simulink model "Marine_LocoMotive_UAV"  (R2018a)
settings: Solver=ode4  StartTime=0.0  StopTime=80  FixedStep=T  RelTol=1e-3
values from neighbouring files (symbols this model uses):
  a_11 = 0.05*m_b    (= 0.625)    [Marine_LocoMotive_UAV.m]
  a_33 = m_b    (= 12.5)    [Marine_LocoMotive_UAV.m]
  A_w = 1*1.5/2    (= 0.75)    [Marine_LocoMotive_UAV.m]
  A_w2 = 1*0.27/2    (= 0.135)    [Marine_LocoMotive_UAV.m]
  Ac = 0.0331    [Marine_LocoMotive_UAV.m]
  alpha_bar = pi/4    (= 0.785398163397)    [Marine_LocoMotive_UAV.m]
  Am = sysd.denominator{1}    [Marine_LocoMotive_UAV.m]
  Am1_LPF = sysd.denominator{1}    [Marine_LocoMotive_UAV.m]
  Am2_LPF = sysd.denominator{1}    [Marine_LocoMotive_UAV.m]
  Am_asw_LPF = sysd.denominator{1}    [Marine_LocoMotive_UAV.m]
  Am_coup_LPF = sysd.denominator{1}    [Marine_LocoMotive_UAV.m]
  Am_rdeL_LPF = sysd.denominator{1}    [Marine_LocoMotive_UAV.m]
  Am_reL_LPF = sysd.denominator{1}    [Marine_LocoMotive_UAV.m]
  Am_rref20_LPF = sysd.denominator{1}    [Marine_LocoMotive_UAV.m]
  Am_rref_LPF = sysd.denominator{1}    [Marine_LocoMotive_UAV.m]
  AmAlpha_LPF = sysd.denominator{1}    [Marine_LocoMotive_UAV.m]
  Amp_sf = 3    [Marine_LocoMotive_UAV.m]
  AmV_LPF = sysd.denominator{1}    [Marine_LocoMotive_UAV.m]
  AmZ_LPF = sysd.denominator{1}    [Marine_LocoMotive_UAV.m]
  b_11 = 0    [Marine_LocoMotive_UAV.m]
  b_33 = 2*m_b*omega_h    (= 27.5578302946)    [Marine_LocoMotive_UAV.m]
  Bm = sysd.numerator{1}    [Marine_LocoMotive_UAV.m]
  Bm1_LPF = sysd.numerator{1}    [Marine_LocoMotive_UAV.m]
  Bm2_LPF = sysd.numerator{1}    [Marine_LocoMotive_UAV.m]
  Bm_asw_LPF = sysd.numerator{1}    [Marine_LocoMotive_UAV.m]
  Bm_coup_LPF = sysd.numerator{1}    [Marine_LocoMotive_UAV.m]
  Bm_rdeL_LPF = sysd.numerator{1}    [Marine_LocoMotive_UAV.m]
  Bm_reL_LPF = sysd.numerator{1}    [Marine_LocoMotive_UAV.m]
  Bm_rref20_LPF = sysd.numerator{1}    [Marine_LocoMotive_UAV.m]
  Bm_rref_LPF = sysd.numerator{1}    [Marine_LocoMotive_UAV.m]
  BmAlpha_LPF = sysd.numerator{1}    [Marine_LocoMotive_UAV.m]
  BmV_LPF = sysd.numerator{1}    [Marine_LocoMotive_UAV.m]
  BmZ_LPF = sysd.numerator{1}    [Marine_LocoMotive_UAV.m]
  C_S = [5;9]*10^-3    [Marine_LocoMotive_UAV.m]
  Cd_u = 0.2    [Marine_LocoMotive_UAV.m]
  D_x = b_11 + D_s(1)    [Marine_LocoMotive_UAV.m]
  D_z = b_33 + D_s(2)    [Marine_LocoMotive_UAV.m]
  dc_M_p = 6.7    [Marine_LocoMotive_UAV.m]
  Delta_h = (A_im/A_b-0.5)*h_b    (= -0.0625)    [Marine_LocoMotive_UAV.m]
  eps_V = 0.1    [Marine_LocoMotive_UAV.m]
  epsilon_1 = 5    [Marine_LocoMotive_UAV.m]
  epsilon_e_u1 = 0.05    [Marine_LocoMotive_UAV.m]
  epsilon_w = 0    [Marine_LocoMotive_UAV.m]
  epsilon_w2 = pi    (= 3.14159265359)    [Marine_LocoMotive_UAV.m]
  g = 9.81    [Marine_LocoMotive_UAV.m]
  gamma_d_p = (2*0.3/0.03*2*0.2*12/4)/10    (= 2.4)    [Marine_LocoMotive_UAV.m]
  H = 10    [Marine_LocoMotive_UAV.m]
  h_b = 0.25    [Marine_LocoMotive_UAV.m]
  J_b = m_b*h_b*l_b/12    (= 0.208333333333)    [Marine_LocoMotive_UAV.m]
  J_u = 0.03    [Marine_LocoMotive_UAV.m]
  K = 40    [Marine_LocoMotive_UAV.m]
  k3 = 24    [Marine_LocoMotive_UAV.m]
  k4 = 0.8    [Marine_LocoMotive_UAV.m]
  k_w = omega_w^2/g    (= 0.123862835563)    [Marine_LocoMotive_UAV.m]
  k_w2 = omega_w2^2/g    (= 0.447144836384)    [Marine_LocoMotive_UAV.m]
  kd_a = 5.6    [Marine_LocoMotive_UAV.m]
  kd_r = 19.5    [Marine_LocoMotive_UAV.m]
  kd_t = 10    [Marine_LocoMotive_UAV.m]
  kd_x = 5    [Marine_LocoMotive_UAV.m]
  kd_z = 2    [Marine_LocoMotive_UAV.m]
  ki_a = 1.6    [Marine_LocoMotive_UAV.m]
  ki_r = 9    [Marine_LocoMotive_UAV.m]
  ki_T = 12    [Marine_LocoMotive_UAV.m]
  ki_x = 1.2    [Marine_LocoMotive_UAV.m]
  ki_z = 1    [Marine_LocoMotive_UAV.m]
  kp_a = 9.6    [Marine_LocoMotive_UAV.m]
  kp_r = 45    [Marine_LocoMotive_UAV.m]
  kp_t = 20    [Marine_LocoMotive_UAV.m]
  kp_T = 25    [Marine_LocoMotive_UAV.m]
  kp_x = 7    [Marine_LocoMotive_UAV.m]
  kp_z = 3    [Marine_LocoMotive_UAV.m]
  L = 0.2    [Marine_LocoMotive_UAV.m]
  l_b = 0.8    [Marine_LocoMotive_UAV.m]
  Lc_0 = 7    [Marine_LocoMotive_UAV.m]
  LIMIT_CMD_PITCH = 45*pi/180    (= 0.785398163397)    [Marine_LocoMotive_UAV.m]
  LIMIT_uCMD_HEIGHT = 3.5*K    (= 140)    [Marine_LocoMotive_UAV.m]
  m_b = rho_w*Vol_b/4    (= 12.5)    [Marine_LocoMotive_UAV.m]
  m_u = 1.8    [Marine_LocoMotive_UAV.m]
  min_sf = 5    [Marine_LocoMotive_UAV.m]
  nu_w = 1.787*10^-6    (= 1.787e-06)    [Marine_LocoMotive_UAV.m]
  omega_w = 2*pi/T_w    (= 1.10231321179)    [Marine_LocoMotive_UAV.m]
  omega_w2 = 2*pi/T_w2    (= 2.09439510239)    [Marine_LocoMotive_UAV.m]
  r_0 = sqrt( (X0_b(1) - X0_u(1))^2 +(X0_b(2) - X0_u(2))^2 )    [Marine_LocoMotive_UAV.m]
  r_bar = Lc_0-0.3    (= 6.7)    [Marine_LocoMotive_UAV.m]
  r_min = (zu_bar-H)-0.2    [Marine_LocoMotive_UAV.m]
  rho_a = 1.225    [Marine_LocoMotive_UAV.m]
  rho_w = 1000    [Marine_LocoMotive_UAV.m]
  T = 1/500    (= 0.002)    [Marine_LocoMotive_UAV.m]
  T_init = 10    [Marine_LocoMotive_UAV.m]
  Theta0 = 0*atan2(V_bar*D_x*cos(alpha_bar_0),V_bar*D_x*sin(alpha_bar_0)+m_u*g*cos(alpha_bar_0))    [Marine_LocoMotive_UAV.m]
  u_s = w_dir*A_w^2*omega_w*k_w*exp(2*k_w*(-Delta_h/2))    [Marine_LocoMotive_UAV.m]
  u_s2 = w_dir2*A_w2^2*omega_w2*k_w2*exp(2*k_w2*(-Delta_h/2))    [Marine_LocoMotive_UAV.m]
  u_t = -1*0.5*1    (= -0.5)    [Marine_LocoMotive_UAV.m]
  u_w = 0*0.2    (= 0)    [Marine_LocoMotive_UAV.m]
  V0_b = [u_t+u_w+u_s+v_x_w, v_z_w]    [Marine_LocoMotive_UAV.m]
  V0_u = [0 0]    [Marine_LocoMotive_UAV.m]
  V_bar = 4    [Marine_LocoMotive_UAV.m]
  Vol_b = A_b*l_b    (= 0.05)    [Marine_LocoMotive_UAV.m]
  w_dir = 1    [Marine_LocoMotive_UAV.m]
  w_dir2 = 1    [Marine_LocoMotive_UAV.m]
  X0_b = [0,H-Delta_h]    [Marine_LocoMotive_UAV.m]
  X0_u = X0_b + [3 3]    [Marine_LocoMotive_UAV.m]
  zu_bar = X0_b(2) + Lc_0*sin(alpha_bar_0)    [Marine_LocoMotive_UAV.m]
undefined symbols (not defined in the file or in its folder): Am_HPF, Am_LPF, Am_LPF2, an1, an1_v, an2, an3, Bm_HPF, Bm_LPF, Bm_LPF2, bn1, bn1_v, bn2, bn3, DiscIntNeverNeededParam, F, Light, magnitude, MIL, OMEGA_FILTER_OUTER, R_b, Tc, Tg, Tn, Ts, Tsc, Tz, X_GPS_offset
libraries: simulink x50, simulink_extras x9, aerolibwind2 x2
(part 4 of 6)

== system Marine_LocoMotive_UAV/Quadrotor+buoy/3-DOF equations of motion Earth frame/M_12 ==
  theta : Inport
  Bias : Bias
  Bias1 : Bias
  Signal Specification1 : SignalSpecification  Dimensions=2
  Signal Specification2 : SignalSpecification  Dimensions=2
  Vector Concatenate1 : Concatenate  Mode=Multidimensional array  ConcatenateDimension=2
  Vector Concatenate2 : Concatenate
  Vector Concatenate3 : Concatenate
  added mass : Subsystem
  M_12 : Outport
  wires:
  Signal Specification2/1 -> Vector Concatenate1/2
  Signal Specification1/1 -> Vector Concatenate1/1
  Vector Concatenate1/1 -> M_12/1
  Bias1/1 -> Vector Concatenate3/2
  Bias/1 -> Vector Concatenate2/1
  added mass/2(M22_I) -> Bias1/1
  added mass/3(M12_I) -> Vector Concatenate2/2, Vector Concatenate3/1
  Vector Concatenate2/1 -> Signal Specification1/1
  added mass/1(M11_I) -> Bias/1
  Vector Concatenate3/1 -> Signal Specification2/1
  theta/1 -> added mass/1(theta)

== system Marine_LocoMotive_UAV/Quadrotor+buoy/3-DOF equations of motion Earth frame/M_123 ==
  theta : Inport
  alpha : Inport  Port=2
  coupled : Inport  Port=3
  Constant1 : Constant  Value=m_u*L^2
  Constant2 : Constant  Value=m_u
  Gain : Gain  Gain=-L
  Gain1 : Gain  Gain=L
  Gain2 : Gain  Gain=L^2
  Product : Product
  Product1 : Product
  Product2 : Product
  Signal Specification1 : SignalSpecification  Dimensions=3
  Signal Specification2 : SignalSpecification  Dimensions=3
  Signal Specification3 : SignalSpecification  Dimensions=3
  Sum : Sum  Inputs=++|
  Sum1 : Sum  Inputs=++|
  Switch : Switch  Criteria=u2 > Threshold
  T, r,xu,xb{1..7} (7 alike) : Scope
  Trigonometric Function : Trigonometry  Operator=sincos
  Vector Concatenate1 : Concatenate  NumInputs=3  Mode=Multidimensional array  ConcatenateDimension=2
  Vector Concatenate2 : Concatenate  NumInputs=3
  Vector Concatenate3 : Concatenate  NumInputs=3
  Vector Concatenate4 : Concatenate  NumInputs=3
  buoy inertia : Subsystem
  M_123 : Outport
  wires:
  theta/1 -> buoy inertia/1(theta)
  Vector Concatenate3/1 -> Signal Specification2/1
  buoy inertia/1(M11_I) -> Sum/2
  Vector Concatenate2/1 -> "T, r,xu,xb7"/1, Signal Specification1/1
  Vector Concatenate4/1 -> "T, r,xu,xb6"/1, Signal Specification3/1
  buoy inertia/3(M12_I) -> Vector Concatenate2/2, Vector Concatenate3/1
  Gain/1 -> "T, r,xu,xb3"/1, Vector Concatenate4/1, Vector Concatenate2/3
  buoy inertia/2(M22_I) -> Sum1/2
  Sum/1 -> Vector Concatenate2/1
  Sum1/1 -> Vector Concatenate3/2
  alpha/1 -> Trigonometric Function/1
  Product1/1 -> Gain/1
  Product2/1 -> Gain1/1
  Switch/1 -> "T, r,xu,xb5"/1, Vector Concatenate4/3
  Vector Concatenate1/1 -> M_123/1
  Signal Specification1/1 -> Vector Concatenate1/1
  Signal Specification2/1 -> Vector Concatenate1/2
  Signal Specification3/1 -> Vector Concatenate1/3
  coupled/1 -> Switch/2, Product/2, "T, r,xu,xb1"/1
  Constant2/1 -> Product/1
  Trigonometric Function/1 -> Product1/2
  Trigonometric Function/2 -> Product2/2
  Gain1/1 -> "T, r,xu,xb4"/1, Vector Concatenate4/2, Vector Concatenate3/3
  Product/1 -> Gain2/1, Product2/1, Product1/1, "T, r,xu,xb2"/1, Sum/1, Sum1/1
  Gain2/1 -> Switch/1
  Constant1/1 -> Switch/3

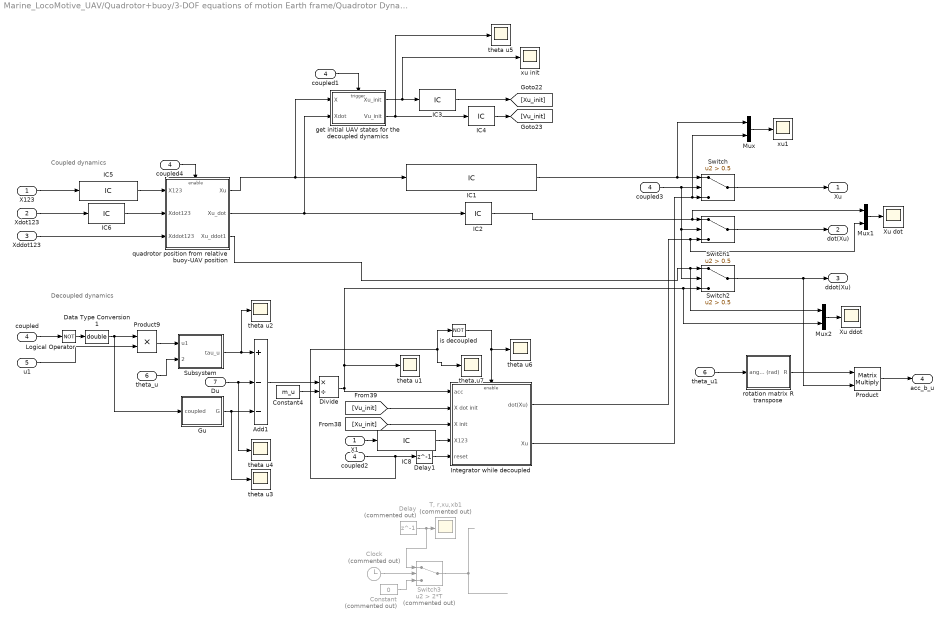
== system Marine_LocoMotive_UAV/Quadrotor+buoy/3-DOF equations of motion Earth frame/Quadrotor Dynamics Outer-Loop ==
  note: Decoupled dynamics
  note: Coupled dynamics
  X123 : Inport
  Xdot123 : Inport  Port=2
  Xddot123 : Inport  Port=3
  coupled : Inport  Port=4
  u1 : Inport  Port=5
  theta_u : Inport  Port=6
  Du : Inport  Port=7
  Add1 : Sum  Inputs=+--
  Clock : Clock  Commented=on
  Constant : Constant  Commented=on  Value=0
  Constant4 : Constant  Value=m_u
  Data Type Conversion1 : DataTypeConversion  OutDataTypeStr=double
  Delay : Delay  Commented=on  DelayLength=1
  Delay1 : Delay  DelayLength=1
  Divide : Product  Inputs=*/
  Gu : Subsystem
  IC1 : InitialCondition  Value=pos_b_ini+L*[cos(alpha_0) sin(alpha_0)]
  IC2 : InitialCondition  Value=[0 0]
  IC3 : InitialCondition  Value=X0_u
  IC4 : InitialCondition  Value=[0 0]
  IC5 : InitialCondition  Value=[X0_b alpha_bar]
  IC6 : InitialCondition  Value=[v_b_ini 0]
  IC8 : InitialCondition  Value=[X0_b alpha_bar]
  Integrator while decoupled : Subsystem  TreatAsAtomicUnit=on
  Logical Operator : Logic  Operator=NOT  AllPortsSameDT=off
  Mux : Mux  Inputs=2
  Mux1 : Mux  Inputs=2
  Mux2 : Mux  Inputs=2
  Product : Product  Multiplication=Matrix(*)
  Product9 : Product  Inputs=**  SaturateOnIntegerOverflow=on  InputSameDT=on  OutDataTypeStr=Inherit: Same as first input
  Subsystem : Subsystem
  Switch : Switch  Criteria=u2 > Threshold  Threshold=0.5
  Switch1 : Switch  Criteria=u2 > Threshold  Threshold=0.5
  Switch2 : Switch  Criteria=u2 > Threshold  Threshold=0.5
  Switch3 : Switch  Commented=on  Criteria=u2 > Threshold  Threshold=2*T
  "T, r,xu,xb1" : Scope  Commented=on
  X1 : InportShadow
  "Xu ddot  " : Scope
  "Xu dot " : Scope
  coupled{1..4} (4 alike) : InportShadow  Port=4
  get initial UAV states for the decoupled dynamics : Subsystem  TreatAsAtomicUnit=on
  is decoupled : Logic  Operator=NOT  AllPortsSameDT=off
  quadrotor position from relative buoy-UAV position : Subsystem
  rotation matrix R transpose : Subsystem
  theta u{1..7} (7 alike) : Scope
  theta_u1 : InportShadow  Port=6
  xu init : Scope
  xu1 : Scope
  Xu : Outport
  dot(Xu) : Outport  Port=2
  ddot(Xu) : Outport  Port=3
  acc_b_u : Outport  Port=4
  wires:
  Subsystem/1(tau_u) -> theta u2/1, Add1/1
  Product9/1 -> Subsystem/1(u1)
  Gu/1(G) -> theta u3/1, Add1/3
  X123/1 -> IC5/1
  Data Type Conversion1/1 -> Product9/1, Gu/1(coupled)
  Add1/1 -> Divide/1
  Logical Operator/1 -> Data Type Conversion1/1
  get initial UAV states for the decoupled dynamics/1(Xu_init) -> xu init/1, IC3/1
  get initial UAV states for the decoupled dynamics/2(Vu_init) -> IC4/1, theta u5/1
  Constant4/1 -> Divide/2
  theta_u/1 -> Subsystem/2(theta_u)
  coupled1/1 -> get initial UAV states for the decoupled dynamics/Trigger
  Du/1 -> Add1/2, theta u4/1
  coupled/1 -> Logical Operator/1
  u1/1 -> Product9/2
  coupled3/1 -> Switch2/2, Switch1/2, Switch/2
  Integrator while decoupled/2("Xu ") -> Mux/2, Switch/3
  quadrotor position from relative buoy-UAV position/1(Xu) -> IC1/1, get initial UAV states for the decoupled dynamics/1(X)
  Mux/1 -> xu1/1
  Mux1/1 -> "Xu dot "/1
  Integrator while decoupled/1("dot(Xu) ") -> Mux1/2, Switch1/3
  Mux2/1 -> "Xu ddot  "/1
  Divide/1 -> Mux2/2, Switch2/3, theta u1/1, Integrator while decoupled/1(acc)
  Switch2/1 -> Product/2, ddot(Xu)/1
  Xdot123/1 -> IC6/1
  Xddot123/1 -> quadrotor position from relative buoy-UAV position/3(Xddot123)
  quadrotor position from relative buoy-UAV position/2(Xu_dot) -> get initial UAV states for the decoupled dynamics/2(Xdot), IC2/1
  quadrotor position from relative buoy-UAV position/3(Xu_ddot1) -> Mux2/1, Switch2/1
  is decoupled/1 -> theta u6/1, Integrator while decoupled/Enable
  coupled2/1 -> Delay1/1, is decoupled/1, theta u7/1
  Switch1/1 -> dot(Xu)/1
  coupled4/1 -> quadrotor position from relative buoy-UAV position/Enable
  Switch/1 -> Xu/1
  Constant/1 -> Switch3/3
  ? -> Delay/1
  Switch3/1 -> ?
  Delay/1 -> Switch3/1, "T, r,xu,xb1"/1
  Clock/1 -> Switch3/2
  [Vu_init] -> Integrator while decoupled/2(X dot init)
  [Xu_init] -> Integrator while decoupled/3(X init)
  X1/1 -> IC8/1
  Delay1/1 -> Integrator while decoupled/5(reset)
  IC3/1 -> [Xu_init]
  IC4/1 -> [Vu_init]
  IC1/1 -> Mux/1, Switch/1
  IC2/1 -> Mux1/1, Switch1/1
  IC5/1 -> quadrotor position from relative buoy-UAV position/1(X123)
  IC8/1 -> Integrator while decoupled/4(X123)
  IC6/1 -> quadrotor position from relative buoy-UAV position/2(Xdot123)
  theta_u1/1 -> rotation matrix R transpose/1(angle (rad))
  rotation matrix R transpose/1(R) -> Product/1
  Product/1 -> acc_b_u/1

== system Marine_LocoMotive_UAV/Quadrotor+buoy/3-DOF equations of motion Earth frame/Tension from Buoy, X direction ==
  alpha : Inport
  M12 : Inport  Port=2
  D12 : Inport  Port=3
  Vr,Wr : Inport  Port=4
  Xb_ddot : Inport  Port=5
  G : Inport  Port=6
  FB : Inport  Port=7
  Add1 : Sum  Inputs=+++-
  Constant : Constant  Value=0
  Math Function : Math  Operator=reciprocal  SaturateOnIntegerOverflow=on
  Math Function1 : Math  Operator=reciprocal  SaturateOnIntegerOverflow=on
  Product1 : Product
  Product2 : Product  Inputs=**  Multiplication=Matrix(*)
  Product3 : Product  Inputs=**  Multiplication=Matrix(*)
  Scope5 : Scope
  Trigonometric Function3 : Trigonometry  Operator=sincos
  Vector Concatenate2 : Concatenate
  Vector Concatenate3 : Concatenate
  T x,z : Outport
  wires:
  alpha/1 -> Trigonometric Function3/1
  M12/1 -> Product2/1
  Vr,Wr/1 -> Product3/2
  D12/1 -> Product3/1
  Xb_ddot/1 -> Product2/2
  G/1 -> Add1/3
  Product2/1 -> Add1/2
  Trigonometric Function3/2 -> Math Function/1
  Trigonometric Function3/1 -> Math Function1/1
  Product3/1 -> Add1/1
  Math Function/1 -> Vector Concatenate2/1
  Math Function1/1 -> Vector Concatenate2/2
  Constant/1 -> Vector Concatenate3/1
  Vector Concatenate3/1 -> Add1/4
  FB/1 -> Vector Concatenate3/2
  Product1/1 -> Scope5/1, T x,z/1
  Vector Concatenate2/1 -> Product1/2
  Add1/1 -> Product1/1

== system Marine_LocoMotive_UAV/Quadrotor+buoy/3-DOF equations of motion Earth frame/Tension from UAV, X and r directions ==
  alpha : Inport
  r_p_ddot : Inport  Port=2
  theta_u : Inport  Port=3
  u1 : Inport  Port=4
  Xb_ddot : Inport  Port=5
  Xu_ddot : Inport  Port=6
  Add1 : Sum  Inputs=+-+
  Add2 : Sum  Inputs=---
  Add3 : Sum  Commented=on  Inputs=+-
  Discrete Derivative2 : simulink/Discrete/Discrete Derivative  Commented=on  gainval=1.0  ICPrevScaledInput=L*500  OutMin=[]  OutMax=[]  OutDataType=fixdt(1, 16)  OutScaling=2^-10  DoSatur=off
  Discrete Derivative3 : simulink/Discrete/Discrete Derivative  Commented=on  gainval=1.0  ICPrevScaledInput=0  OutMin=[]  OutMax=[]  OutDataType=fixdt(1, 16)  OutScaling=2^-10  DoSatur=off
  Gain14 : Gain  Commented=on
  Gain15 : Gain  Commented=on  Gain=m_u
  Gain5 : Gain  Gain=m_u
  Gain6 : Gain  Gain=m_u*g
  Product10 : Product  Inputs=**  Multiplication=Matrix(*)
  Product12 : Product  Commented=on
  Product7 : Product
  Product9 : Product  Commented=on  Inputs=*/
  Signal Specification{1,4..6} (4 alike) : SignalSpecification  Dimensions=1
  Signal Specification2 : SignalSpecification  Dimensions=[1,2]
  Sum4 : Sum  Inputs=|++
  "T, r,xu,xb1" : Scope
  "T, r,xu,xb2" : Scope
  "T, r,xu,xb3" : Scope
  "Tension from UAV, X and r directions" : Subsystem
  Trigonometric Function2 : Trigonometry
  Trigonometric Function3 : Trigonometry  Operator=sincos
  Trigonometric Function6 : Trigonometry  Commented=on  Operator=cos
  Trigonometric Function8 : Trigonometry  Commented=on
  Vector Concatenate : Concatenate
  Xu_ddot1 : InportShadow  Port=6
  alpha1 : InportShadow
  r : Constant  Commented=on  Value=L
  theta_u1 : InportShadow  Port=3
  "u1 " : InportShadow  Port=4
  x_ddot1 : Selector  Commented=on  InputPortWidth=2  IndexOptions=Index vector (dialog)  Indices=1  OutputSizes=1
  "T, from r" : Outport
  "T, from uav z" : Outport  Port=2
  wires:
  r/1 -> Discrete Derivative2/1
  r_p_ddot/1 -> Add2/1
  alpha/1 -> Trigonometric Function3/1
  Sum4/1 -> Trigonometric Function2/1
  [alpha] -> Sum4/1
  u1/1 -> Product7/2
  Add2/1 -> Gain5/1
  Trigonometric Function2/1 -> Product7/1
  Discrete Derivative2/1 -> Discrete Derivative3/1
  Trigonometric Function3/1 -> Signal Specification5/1, Vector Concatenate/2
  Product10/1 -> Add2/2
  Gain5/1 -> "T, r,xu,xb1"/1, Add1/1
  theta_u/1 -> Sum4/2
  Gain6/1 -> "T, r,xu,xb2"/1, Add1/2
  Trigonometric Function3/2 -> Vector Concatenate/1
  Add3/1 -> Product9/1
  Gain14/1 -> Add3/1
  Trigonometric Function8/1 -> Product12/1
  "u1 "/1 -> "Tension from UAV, X and r directions"/3(u1), Product12/2
  alpha1/1 -> "Tension from UAV, X and r directions"/1(alpha), Trigonometric Function6/1
  Product12/1 -> Gain14/1
  x_ddot1/1 -> Gain15/1
  Trigonometric Function6/1 -> Product9/2
  Xu_ddot/1 -> x_ddot1/1
  theta_u1/1 -> "Tension from UAV, X and r directions"/2(theta_u), Trigonometric Function8/1
  Gain15/1 -> Add3/2
  Product7/1 -> Signal Specification6/1
  Signal Specification2/1 -> Product10/1
  Discrete Derivative3/1 -> Signal Specification4/1
  Add1/1 -> Signal Specification1/1
  Vector Concatenate/1 -> Product10/2
  Signal Specification4/1 -> Add2/3
  Signal Specification5/1 -> Gain6/1
  Signal Specification6/1 -> "T, r,xu,xb3"/1, Add1/3
  Xb_ddot/1 -> Signal Specification2/1
  Signal Specification1/1 -> "T, from r"/1
  Xu_ddot1/1 -> "Tension from UAV, X and r directions"/4(Xu_ddot)
  "Tension from UAV, X and r directions"/1("T, from x simple") -> "T, from uav z"/1

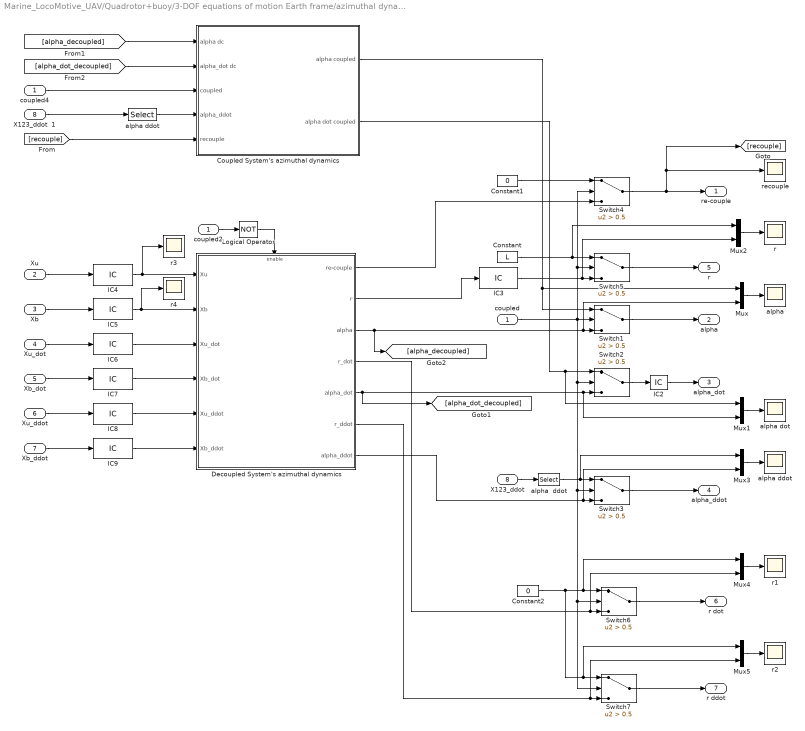
== system Marine_LocoMotive_UAV/Quadrotor+buoy/3-DOF equations of motion Earth frame/azimuthal dynamics ==
  coupled : Inport
  Xu : Inport  Port=2
  Xb : Inport  Port=3
  "Xu_dot " : Inport  Port=4
  Xb_dot : Inport  Port=5
  Xu_ddot : Inport  Port=6
  "Xb_ddot   " : Inport  Port=7
  "X123_ddot  " : Inport  Port=8
  "    alpha ddot" : Scope
  "  alpha" : Scope
  "  alpha dot" : Scope
    r{,1..4} (5 alike) : Scope
  "  recouple   " : Scope
  Constant : Constant  Value=L
  Constant1 : Constant  Value=0
  Constant2 : Constant  Value=0
  Coupled System's azimuthal dynamics : Subsystem
  Decoupled System's azimuthal dynamics : Subsystem  TreatAsAtomicUnit=on
  IC2 : InitialCondition  Value=0
  IC3 : InitialCondition  Value=r_0
  IC4 : InitialCondition  Value=X0_u
  IC5 : InitialCondition  Value=X0_b
  IC6 : InitialCondition  Value=[0 0]
  IC7 : InitialCondition  Value=V0_b
  IC8 : InitialCondition  Value=[0 0]
  IC9 : InitialCondition  Value=[0 0]
  Logical Operator : Logic  Operator=NOT  AllPortsSameDT=off  OutDataTypeStr=boolean
  Mux{,1..5} (6 alike) : Mux  Inputs=2
  Switch{1..7} (7 alike) : Switch  Criteria=u2 > Threshold  Threshold=0.5
  X123_ddot  1 : InportShadow  Port=8
  alpha  ddot : Selector  InputPortWidth=3  IndexOptions=Index vector (dialog)  Indices=3  OutputSizes=1
  alpha ddot : Selector  InputPortWidth=3  IndexOptions=Index vector (dialog)  Indices=3  OutputSizes=1
  coupled2 : InportShadow
  coupled4 : InportShadow
  re-couple : Outport
  alpha : Outport  Port=2
  "alpha_dot " : Outport  Port=3
  alpha_ddot : Outport  Port=4
  "r " : Outport  Port=5
  r dot : Outport  Port=6
  r ddot : Outport  Port=7
  wires:
  coupled/1 -> Switch7/2, Switch6/2, Switch3/2, Switch2/2, Switch4/2, Switch5/2, Switch1/2
  "X123_ddot  "/1 -> alpha  ddot/1
  Switch3/1 -> alpha_ddot/1
  Coupled System's azimuthal dynamics/2(alpha dot coupled) -> Switch2/1, Mux1/1
  Switch2/1 -> IC2/1
  Xb/1 -> IC5/1
  Xu/1 -> IC4/1
  alpha ddot/1 -> Coupled System's azimuthal dynamics/4(alpha_ddot)
  [alpha_dot_decoupled] -> Coupled System's azimuthal dynamics/2(alpha_dot dc)
  coupled4/1 -> Coupled System's azimuthal dynamics/3(coupled)
  [alpha_decoupled] -> Coupled System's azimuthal dynamics/1(alpha dc)
  X123_ddot  1/1 -> alpha ddot/1
  "Xu_dot "/1 -> IC6/1
  Xb_dot/1 -> IC7/1
  "Xb_ddot   "/1 -> IC9/1
  Xu_ddot/1 -> IC8/1
  coupled2/1 -> Logical Operator/1
  Switch5/1 -> "r "/1
  Constant/1 -> Switch5/1, Mux2/1
  Decoupled System's azimuthal dynamics/2(r) -> IC3/1
  [recouple] -> Coupled System's azimuthal dynamics/5(recouple)
  Coupled System's azimuthal dynamics/1(alpha coupled) -> Mux/1, Switch1/1
  Decoupled System's azimuthal dynamics/7(alpha_ddot) -> Mux3/2, Switch3/3
  Logical Operator/1 -> Decoupled System's azimuthal dynamics/Enable
  Mux/1 -> "  alpha"/1
  Mux1/1 -> "  alpha dot"/1
  Decoupled System's azimuthal dynamics/5(alpha_dot) -> Mux1/2, Switch2/3, [alpha_dot_decoupled]
  Mux2/1 -> "  r"/1
  Decoupled System's azimuthal dynamics/1(re-couple) -> Switch4/3
  Mux3/1 -> "    alpha ddot"/1
  alpha  ddot/1 -> Mux3/1, Switch3/1
  Switch4/1 -> [recouple], "  recouple   "/1, re-couple/1
  Constant1/1 -> Switch4/1
  Switch1/1 -> alpha/1
  IC2/1 -> "alpha_dot "/1
  Mux4/1 -> "  r1"/1
  Switch6/1 -> r dot/1
  Decoupled System's azimuthal dynamics/4(r_dot) -> Mux4/2, Switch6/3
  Decoupled System's azimuthal dynamics/6(r_ddot) -> Switch7/3, Mux5/2
  Constant2/1 -> Switch7/1, Mux5/1, Mux4/1, Switch6/1
  Switch7/1 -> r ddot/1
  Mux5/1 -> "  r2"/1
  IC3/1 -> Mux2/2, Switch5/3
  IC4/1 -> "  r3"/1, Decoupled System's azimuthal dynamics/1(Xu)
  IC6/1 -> Decoupled System's azimuthal dynamics/3(Xu_dot)
  IC7/1 -> Decoupled System's azimuthal dynamics/4(Xb_dot)
  IC8/1 -> Decoupled System's azimuthal dynamics/5(Xu_ddot)
  IC9/1 -> Decoupled System's azimuthal dynamics/6(Xb_ddot)
  Decoupled System's azimuthal dynamics/3(alpha) -> Switch1/3, Mux/2, [alpha_decoupled]
  IC5/1 -> "  r4"/1, Decoupled System's azimuthal dynamics/2(Xb)

== system Marine_LocoMotive_UAV/Quadrotor+buoy/3-DOF equations of motion Earth frame/buoyancy ==
  z_b : Inport
  zeta : Inport  Port=2
  Constant : Constant  Commented=on  Value=g*rho_w*l_b*R_b
  Manual Switch : ManualSwitch  CurrentSetting=0
  Product : Product  Commented=on
  Scope1 : Scope  Commented=on
  Scope3 : Scope  Commented=on
  V_im cuboid : Subsystem
  f(z_b,zeta) cylinder : Subsystem  Commented=on
  two connected cylindrical buoys : Gain  Commented=on  Gain=2
  two connected cylindrical buoys1 : Gain  Commented=on  Gain=l_b*R_b
  two connected cylindrical buoys2 : Gain  Commented=on  Gain=2
  V_im : Outport
  wires:
  z_b/1 -> V_im cuboid/2(zb), f(z_b,zeta) cylinder/2(zb)
  zeta/1 -> V_im cuboid/1(zeta), f(z_b,zeta) cylinder/1(zeta)
  Product/1 -> two connected cylindrical buoys/1
  Constant/1 -> Scope1/1, Product/2
  f(z_b,zeta) cylinder/1(Out1) -> two connected cylindrical buoys1/1, Product/1, Scope3/1
  Manual Switch/1 -> V_im/1
  V_im cuboid/1(Vol_im) -> Manual Switch/2
  two connected cylindrical buoys1/1 -> two connected cylindrical buoys2/1
  two connected cylindrical buoys2/1 -> Manual Switch/1

== system Marine_LocoMotive_UAV/Quadrotor+buoy/3-DOF equations of motion Earth frame/rotation matrix R  ==
  angle (rad) : Inport
  Gain : Gain  Gain=-1
  Signal Specification1 : SignalSpecification  Dimensions=2
  Signal Specification2 : SignalSpecification  Dimensions=2
  Trigonometric Function1 : Trigonometry  Operator=sincos
  Vector Concatenate1 : Concatenate  Mode=Multidimensional array  ConcatenateDimension=2
  Vector Concatenate2 : Concatenate
  Vector Concatenate3 : Concatenate
  R : Outport
  wires:
  Signal Specification2/1 -> Vector Concatenate1/2
  Signal Specification1/1 -> Vector Concatenate1/1
  Vector Concatenate1/1 -> R/1
  Vector Concatenate2/1 -> Signal Specification1/1
  Vector Concatenate3/1 -> Signal Specification2/1
  angle (rad)/1 -> Trigonometric Function1/1
  Trigonometric Function1/2 -> Vector Concatenate3/2, Vector Concatenate2/1
  Trigonometric Function1/1 -> Vector Concatenate2/2, Gain/1
  Gain/1 -> Vector Concatenate3/1

== system Marine_LocoMotive_UAV/Quadrotor+buoy/3-DOF equations of motion Earth frame/u123 ==
  u1 : Inport
  theta : Inport  Port=2
  V_im : Inport  Port=3
  alpha : Inport  Port=4
  coupled : Inport  Port=5
  Constant1 : Constant  Value=rho_w*g
  Constant2 : Constant  Commented=on  Value=Vol_b/2
  F_B : Product
  Gain : Gain  Gain=L
  Product1 : Product  Inputs=3  SaturateOnIntegerOverflow=on  InputSameDT=on  OutDataTypeStr=Inherit: Same as first input
  Product2 : Product  Inputs=**  SaturateOnIntegerOverflow=on  InputSameDT=on  OutDataTypeStr=Inherit: Same as first input
  Product6 : Product  Inputs=**  SaturateOnIntegerOverflow=on  InputSameDT=on  OutDataTypeStr=Inherit: Same as first input
  Product7 : Product  Inputs=**  SaturateOnIntegerOverflow=on  InputSameDT=on  OutDataTypeStr=Inherit: Same as first input
  Scope9 : Scope
  Signal Specification2 : SignalSpecification  Dimensions=3
  Sum1 : Sum  Inputs=|++  SaturateOnIntegerOverflow=on
  Sum2 : Sum  Inputs=|++  SaturateOnIntegerOverflow=on
  Trigonometric Function1 : Trigonometry  Operator=sincos
  Trigonometric Function2 : Trigonometry  Operator=cos
  Vector Concatenate3 : Concatenate  NumInputs=3
  coupled1 : InportShadow  Port=5
  u2 : InportShadow
  u123 : Outport
  wires:
  Product7/1 -> Sum1/1
  Product2/1 -> Product7/2, Product6/1
  Trigonometric Function1/2 -> Product7/1
  Product1/1 -> Vector Concatenate3/3
  Vector Concatenate3/1 -> Scope9/1, Signal Specification2/1
  Product6/1 -> Vector Concatenate3/1
  Sum1/1 -> Vector Concatenate3/2
  Trigonometric Function1/1 -> Product6/2
  F_B/1 -> Sum1/2
  theta/1 -> Sum2/1, Trigonometric Function1/1
  V_im/1 -> F_B/1
  alpha/1 -> Sum2/2
  Sum2/1 -> Trigonometric Function2/1
  Trigonometric Function2/1 -> Gain/1
  Gain/1 -> Product1/2
  u2/1 -> Product1/1
  Constant1/1 -> F_B/2
  Signal Specification2/1 -> u123/1
  coupled/1 -> Product2/1
  u1/1 -> Product2/2
  coupled1/1 -> Product1/3

== system Marine_LocoMotive_UAV/Sensors and Filters/Coupling detection by r/Coupling state ==
  r_est : Inport
  re_couple : Inport  Port=2
  Data Type Conversion : DataTypeConversion  OutDataTypeStr=double
  Delay10 : Delay  DelayLength=1  InitialCondition=0
  IC3 : InitialCondition  Value=0
  IC5 : InitialCondition  Value=0
  MATLAB Function : MATLAB Function  TreatAsAtomicUnit=on
  "T, r,xu,xb1" : Scope
  break algebraic loop : Delay  DelayLength=1  InitialCondition=1
  cable length with safety margine1 : simulink/Logic and Bit Operations/Compare To Constant  relop=>=  const=Lc_0-0.05  OutDataTypeStr=boolean
  "is coupled " : Scope
  is coupled -1 : Scope
  pos tension : Scope
  positive tension : Scope
  "re_couple " : Scope
  state detector : Scope
  is coupled : Outport
  wires:
  Delay10/1 -> is coupled -1/1, MATLAB Function/3(coupled)
  IC5/1 -> is coupled/1, Delay10/1
  MATLAB Function/1(is_coupled) -> IC5/1, "is coupled "/1
  break algebraic loop/1 -> pos tension/1, MATLAB Function/1(pos_T)
  re_couple/1 -> MATLAB Function/2(re_couple), "re_couple "/1
  MATLAB Function/2(c) -> state detector/1
  Data Type Conversion/1 -> positive tension/1, break algebraic loop/1
  IC3/1 -> Data Type Conversion/1
  cable length with safety margine1/1 -> IC3/1
  r_est/1 -> "T, r,xu,xb1"/1, cable length with safety margine1/1

== system Marine_LocoMotive_UAV/Sensors and Filters/Data processing/Estimate Attitude ==
  Acc : Inport
  q : Inport  Port=2
  Euler : Inport  Port=3
  Calculate Roll and Pitch (From Acceleration Data) : Subsystem
  Constant : Constant  Value=Ts
  Demux : Demux  Outputs=2
  Ground : Ground
  High Pass Filter1 : DiscreteTransferFcn  Numerator=Bm_HPF  Denominator=Am_HPF
  Kalman Filter - Pitch : MATLAB Function  TreatAsAtomicUnit=on
  Manual Switch1 : ManualSwitch  CurrentSetting=0
  Mux : Mux  Inputs=3
  Mux2 : Mux  Inputs=2
  Mux5 : Mux  Inputs=2
  Notch Filter1 : Subsystem
  Scope1 : Scope
  Signal Specification : SignalSpecification  Dimensions=1
  theta : Scope
  q_g : Outport
  q_f : Outport  Port=2
  " pitch" : Outport  Port=3
  wires:
  q/1 -> High Pass Filter1/1, Mux2/2
  Notch Filter1/2(q) -> Kalman Filter - Pitch/2(gyro_rate), q_f/1
  Calculate Roll and Pitch (From Acceleration Data)/1(pitch_acc (rad)) -> Kalman Filter - Pitch/1(acc_angle)
  Signal Specification/1 -> " pitch"/1  "Kalman"
  Euler/1 -> Mux5/1, Kalman Filter - Pitch/3(opti_angle)  "pitch"
  Constant/1 -> Kalman Filter - Pitch/4(dt)
  Acc/1 -> Demux/1
  Notch Filter1/1(y) -> Manual Switch1/2
  High Pass Filter1/1 -> Manual Switch1/1, Notch Filter1/1(u), Mux2/1
  Mux2/1 -> Scope1/1
  Kalman Filter - Pitch/1(angle) -> Mux5/2, Signal Specification/1
  Mux/1 -> Calculate Roll and Pitch (From Acceleration Data)/1(accel (m/s^2) [3])
  Demux/1 -> Mux/1
  Demux/2 -> Mux/3
  Ground/1 -> Mux/2
  Manual Switch1/1 -> q_g/1
  Mux5/1 -> theta/1

== system Marine_LocoMotive_UAV/Sensors and Filters/Data processing/Estimate Position ==
  OptiTrack : Inport
  "pitch, Kalman" : Inport  Port=2
  Sonar : Inport  Port=3
  2nd Order Filter : Subsystem
  2nd Order Filter2 : Subsystem
  2nd Order Filter4 : Subsystem
  2nd Order Filter5 : Subsystem
  Constant4 : Constant  Value=Tc
  Demux2 : Demux
  Extrapolation - x : MATLAB Function  TreatAsAtomicUnit=on
  Extrapolation - z : MATLAB Function  TreatAsAtomicUnit=on
  Height est : Scope
  Height est1 : Scope
  Kalman Filter - Height : MATLAB Function  TreatAsAtomicUnit=on
  Manual Switch : ManualSwitch  CurrentSetting=0
  Mux : Mux  Inputs=2
  Mux1 : Mux  Inputs=2
  Mux2 : Mux  Inputs=3
  Mux3 : Mux  Inputs=3
  Mux4 : Mux  Inputs=3
  Notch Filter2 : Subsystem
  Position : Selector  InputPortWidth=5  IndexOptions=Index vector (dialog)  Indices=[1 2 4 5]  OutputSizes=1
  Signal Conditioning - Sonar : Subsystem
  Signal Specification : SignalSpecification  Dimensions=2
  Signal Specification1 : SignalSpecification  Dimensions=2
  Step Size : Constant  Value=Tc
  Step Size1 : Constant  Value=X0_u(1)
  Step Size2 : Constant  Value=X0_u(2)
  Step Size3 : Constant  Value=X0_u(2)
  Terminator1 : Terminator
  Terminator2 : Terminator
  Thrust1 : Scope
  Thrust11 : Scope
  V_est : Scope  Commented=on
  X_est : Scope  Commented=on
  Xe : Outport
  Ve : Outport  Port=2
  wires:
  Demux2/1 -> Mux3/1, Extrapolation - x/1(xin)
  2nd Order Filter5/2(yd) -> [height_rate_Kalman]
  Demux2/3 -> Extrapolation - x/4(new), Extrapolation - z/4(new)  "New Data"
  Constant4/1 -> Kalman Filter - Height/3(dt)
  Extrapolation - x/1(xout) -> Mux3/2, 2nd Order Filter/1(u)
  2nd Order Filter/1(y) -> Mux3/3, Mux/1
  2nd Order Filter4/2(yd) -> Kalman Filter - Height/2(sonar_d)
  2nd Order Filter2/1(y) -> Mux4/3, Kalman Filter - Height/1(optitrack), Mux2/2
  Sonar/1 -> Signal Conditioning - Sonar/1(sonar (m))
  2nd Order Filter4/1(y) -> Terminator1/1
  Signal Conditioning - Sonar/1(calib sonar (m)) -> Mux2/1, 2nd Order Filter4/1(u)
  Step Size/1 -> Extrapolation - z/3(dt), Extrapolation - x/3(dt)
  Position/1 -> Demux2/1
  Demux2/2 -> Mux4/1, Extrapolation - z/1(xin)
  2nd Order Filter5/1(y) -> Terminator2/1
  Mux/1 -> Signal Specification/1  "Xe IMU or GPS"
  [height_rate_Kalman] -> Mux1/2
  Demux2/4 -> Extrapolation - x/5(isTracking), Extrapolation - z/5(isTracking)  "Is Tracking"
  Mux2/1 -> Height est/1
  Mux1/1 -> Signal Specification1/1  "Ve IMU or GPS"
  OptiTrack/1 -> Thrust1/1, Position/1
  Mux3/1 -> Thrust11/1
  2nd Order Filter2/2(yd) -> Extrapolation - z/2(xdotin)
  Notch Filter2/1(y) -> Manual Switch/2
  2nd Order Filter/2(yd) -> Notch Filter2/1(u), Manual Switch/1, Extrapolation - x/2(xdotin)
  Manual Switch/1 -> Mux1/1
  Signal Specification/1 -> Xe/1, X_est/1
  Signal Specification1/1 -> Ve/1, V_est/1
  Kalman Filter - Height/1(height) -> [height_Kalman], Mux2/3, 2nd Order Filter5/1(u)
  [height_Kalman] -> Mux/2
  "pitch, Kalman"/1 -> Signal Conditioning - Sonar/2(pitch (rad))
  Mux4/1 -> Height est1/1
  Extrapolation - z/1(xout) -> Mux4/2, 2nd Order Filter2/1(u)
  Step Size1/1 -> Extrapolation - x/6(x0)
  Step Size2/1 -> Extrapolation - z/6(x0)
  Step Size3/1 -> Kalman Filter - Height/4(x0)

== system Marine_LocoMotive_UAV/Sensors and Filters/Sensors/ Sonar (10Hz) (true elevation instead real sonar signal) ==
  note: "Smooth" out the Sonar data
  note: Resample the 10Hz Sonar Data
  sonar (m) : Inport
  FOH1 : Subsystem  mask{Ts=0.1}
      mask prompts: Ts "Sample Time"
  IC : InitialCondition  Value=X0_u(2)
  Rate Transition : RateTransition  InitialCondition=X0_u(2)
  Sampler : Subsystem  mask{Ts=0.1}
      mask prompts: Ts "Sample Time"
  calib sonar (m) : Outport
  wires:
  Sampler/1(Out1) -> Rate Transition/1
  Rate Transition/1 -> FOH1/1(Input)
  sonar (m)/1 -> Sampler/1(In1)
  FOH1/1(Output) -> IC/1
  IC/1 -> calib sonar (m)/1

== system Marine_LocoMotive_UAV/Sensors and Filters/Sensors/Accelerometer (500Hz) ==
  Ab : Inport
  "Ab " : Scope  Commented=on
  Demux1 : Demux  Outputs=2
  From File : FromFile  FileName=acc_x_noise.mat  SampleTime=Tz
  From File2 : FromFile  FileName=acc_z_noise.mat  SampleTime=Tz
  IC : InitialCondition  Value=[0 0]
  Manual Switch{,2,4,6} (4 alike) : ManualSwitch
  Mux1 : Mux  Inputs=2
  Mux2 : Mux  Inputs=2
  Product : Product  SaturateOnIntegerOverflow=on  RndMeth=Zero  InputSameDT=on  OutDataTypeStr=Inherit: Same as first input
  Product2 : Product  SaturateOnIntegerOverflow=on  RndMeth=Zero  InputSameDT=on  OutDataTypeStr=Inherit: Same as first input
  Slider Gain : simulink/Math Operations/Slider Gain  gain=1  low=0  high=2
  Slider Gain2 : simulink/Math Operations/Slider Gain  gain=1  low=0  high=2
  Sum2 : Sum  Inputs=+++  SaturateOnIntegerOverflow=on  InputSameDT=on  OutDataTypeStr=Inherit: Same as first input
  Sum5 : Sum  Inputs=+++  SaturateOnIntegerOverflow=on  InputSameDT=on  OutDataTypeStr=Inherit: Same as first input
  acc_noisy : Scope  Commented=on
  bias : Constant  Value=0.05  VectorParams1D=off
  bias10 : Constant  Value=1.02  VectorParams1D=off
  bias11 : Constant  VectorParams1D=off
  bias3 : Constant  Value=1.02  VectorParams1D=off
  bias4 : Constant  VectorParams1D=off
  bias6 : Constant  Value=0  VectorParams1D=off
  bias7 : Constant  Value=0.05  VectorParams1D=off
  bias8 : Constant  Value=0  VectorParams1D=off
  Acc : Outport
  wires:
  bias11/1 -> Manual Switch6/2
  bias10/1 -> Manual Switch6/1
  bias4/1 -> Manual Switch4/2
  bias3/1 -> Manual Switch4/1
  Manual Switch2/1 -> Sum2/2
  bias8/1 -> Manual Switch2/2
  bias7/1 -> Manual Switch2/1
  bias6/1 -> Manual Switch/2
  bias/1 -> Manual Switch/1
  Manual Switch/1 -> Sum5/2
  Manual Switch6/1 -> Product2/1
  Manual Switch4/1 -> Product/1
  Product2/1 -> Mux1/2
  Sum2/1 -> Product2/2
  Product/1 -> Mux1/1
  Sum5/1 -> Product/2
  From File2/1 -> Slider Gain2/1
  Demux1/1 -> Sum5/3
  Demux1/2 -> Sum2/3
  From File/1 -> Slider Gain/1
  Mux2/1 -> acc_noisy/1
  Mux1/1 -> IC/1
  Ab/1 -> Demux1/1, Mux2/2, "Ab "/1
  Slider Gain/1 -> Sum5/1
  Slider Gain2/1 -> Sum2/1
  IC/1 -> Mux2/1, Acc/1

== system Marine_LocoMotive_UAV/Sensors and Filters/Sensors/GPS (10Hz)  ==
  note: 0.2
  Xe : Inport
  Euler : Inport  Port=2
  DCM_b2e : Inport  Port=3
  Constant : Constant  Value=X_GPS_offset
  Constant1 : Constant
  Demux : Demux  Outputs=2
  IC : InitialCondition  Value=[X0_u Theta0]
  Is Tracking : simulink/Sources/Repeating Sequence Stair  Commented=on  OutValues=[1 1 1 1 1 1 1 1 1 1 1 1 1 1 1 1 1 1 1 1]  tsamp=To  OutMin=[]  OutMax=[]  OutDataTypeStr=double  OutputDataTypeScalingMode=double  OutDataType=fixdt(0,8)  ConRadixGroup=Best Precision: Vector-wise  OutScaling=2^-12
  Logical Operator : Logic  AllPortsSameDT=off  OutDataTypeStr=boolean
  Mux : Mux  Inputs=3
  Mux1 : Mux  Inputs=3
  New Data : simulink/Sources/Repeating Sequence Stair  Commented=on  OutValues=[1 1 1 0 0 1 0 1 1 1 1 0 1 1 0 1 1 1 1 1 0 0 0 1 1 0 1 1 1 0]  tsamp=To  OutMin=[]  OutMax=[]  OutDataTypeStr=double  OutputDataTypeScalingMode=double  OutDataType=fixdt(0,8)  ConRadixGroup=Best Precision: Vector-wise  OutScaling=2^-12
  Product : Product  Multiplication=Matrix(*)
  Random Number : RandomNumber  Variance=5/10000  SampleTime=Tg
  Random Number2 : RandomNumber  Variance=5/10000  SampleTime=Tg
  Random Number4 : RandomNumber  Variance=1/100000  SampleTime=Tg
  Rate Transition : RateTransition
  Rate Transition2 : RateTransition
  Rate Transition4 : RateTransition
  Scope : Scope  Commented=on
  Slider Gain : simulink/Math Operations/Slider Gain  gain=0.5  low=0  high=2
  Slider Gain2 : simulink/Math Operations/Slider Gain  gain=0.5  low=0  high=2
  Slider Gain4 : simulink/Math Operations/Slider Gain  gain=1  low=0  high=2
  Sum : Sum  Inputs=++|
  Sum2 : Sum  Inputs=++|
  Sum4 : Sum  Inputs=++|
  Sum6 : Sum  Inputs=|++
  Switch : Switch  Criteria=u2 > Threshold  Threshold=0.5
  Variable Integer Delay1 : Delay  DelayLength=1
  Variable Integer Delay3 : Delay  DelayLength=1  InitialCondition=[X0_u Theta0]
  optiTrack : Scope  Commented=on
  optiTrack1 : Scope  Commented=on
  optiTrack2 : Scope
  optiTrack3 : Scope
  optiTrack4 : Scope
  GPS : Outport
  wires:
  Mux/1 -> Variable Integer Delay3/1
  Constant1/1 -> Mux1/2, Logical Operator/1, Mux1/3, Logical Operator/2
  Logical Operator/1 -> optiTrack1/1, Switch/2
  Variable Integer Delay1/1 -> Switch/3
  Slider Gain/1 -> Sum2/1
  Random Number2/1 -> Rate Transition2/1
  Demux/1 -> Sum/2
  Demux/2 -> Sum2/2
  Sum2/1 -> Mux/2
  Sum/1 -> Mux/1
  Random Number/1 -> Rate Transition/1
  Slider Gain2/1 -> optiTrack2/1, Sum/1
  Mux1/1 -> GPS/1
  Random Number4/1 -> Rate Transition4/1
  Euler/1 -> Sum4/2
  Sum4/1 -> Mux/3
  Variable Integer Delay3/1 -> Switch/1, optiTrack3/1
  Rate Transition/1 -> Slider Gain2/1
  Rate Transition2/1 -> Scope/1, Slider Gain/1
  Rate Transition4/1 -> Slider Gain4/1
  Switch/1 -> Variable Integer Delay1/1, IC/1  "x,z,theta"
  Sum6/1 -> Demux/1
  DCM_b2e/1 -> Product/1
  Constant/1 -> Product/2
  Product/1 -> Sum6/2
  Xe/1 -> Sum6/1
  IC/1 -> optiTrack/1, Mux1/1
  Slider Gain4/1 -> Sum4/1, optiTrack4/1

== system Marine_LocoMotive_UAV/Sensors and Filters/Sensors/Gyro (500Hz) ==
  q : Inport
  Degrees to Radians2 : simulink_extras/Transformations/Degrees to Radians
  From File1 : FromFile  FileName=gyro_q_noise.mat  SampleTime=Tz
  Manual Switch1 : ManualSwitch
  Manual Switch5 : ManualSwitch  CurrentSetting=0
  Product1 : Product  SaturateOnIntegerOverflow=on  RndMeth=Zero  InputSameDT=on  OutDataTypeStr=Inherit: Same as first input
  Slider Gain1 : simulink/Math Operations/Slider Gain  gain=1  low=0  high=2
  Sum2 : Sum  Inputs=+++  SaturateOnIntegerOverflow=on  InputSameDT=on  OutDataTypeStr=Inherit: Same as first input
  Variable Integer Delay3 : Delay  DelayLength=0
  bias1 : Constant  Value=-1  VectorParams1D=off
  bias2 : Constant  Value=0  VectorParams1D=off
  bias5 : Constant  Value=0.9  VectorParams1D=off
  bias9 : Constant  VectorParams1D=off
  " q" : Outport
  wires:
  bias9/1 -> Manual Switch5/2
  bias5/1 -> Manual Switch5/1
  Manual Switch1/1 -> Degrees to Radians2/1
  bias2/1 -> Manual Switch1/2
  bias1/1 -> Manual Switch1/1
  Degrees to Radians2/1 -> Sum2/2
  Manual Switch5/1 -> Product1/1
  Sum2/1 -> Product1/2
  From File1/1 -> Slider Gain1/1
  Product1/1 -> Variable Integer Delay3/1
  Variable Integer Delay3/1 -> " q"/1
  Slider Gain1/1 -> Sum2/1
  q/1 -> Sum2/3

== system Marine_LocoMotive_UAV/Sensors and Filters/Sensors/rotation matrix R ==
  angle (rad) : Inport
  Gain : Gain  Gain=-1
  Signal Specification1 : SignalSpecification  Dimensions=2
  Signal Specification2 : SignalSpecification  Dimensions=2
  Trigonometric Function1 : Trigonometry  Operator=sincos
  Vector Concatenate1 : Concatenate  Mode=Multidimensional array  ConcatenateDimension=2
  Vector Concatenate2 : Concatenate
  Vector Concatenate3 : Concatenate
  R : Outport
  wires:
  Signal Specification2/1 -> Vector Concatenate1/2
  Signal Specification1/1 -> Vector Concatenate1/1
  Vector Concatenate1/1 -> R/1
  Vector Concatenate2/1 -> Signal Specification1/1
  Vector Concatenate3/1 -> Signal Specification2/1
  angle (rad)/1 -> Trigonometric Function1/1
  Trigonometric Function1/2 -> Vector Concatenate3/2, Vector Concatenate2/1
  Trigonometric Function1/1 -> Vector Concatenate2/2, Gain/1
  Gain/1 -> Vector Concatenate3/1

== system Marine_LocoMotive_UAV/Sensors and Filters/quadrotor position from relative buoy-UAV position/rotation matrix R  ==
  angle (rad) : Inport
  Gain2 : Gain  Gain=-1
  Signal Specification1 : SignalSpecification  Dimensions=2
  Signal Specification2 : SignalSpecification  Dimensions=2
  Trigonometric Function1 : Trigonometry  Operator=sincos
  Vector Concatenate1 : Concatenate  Mode=Multidimensional array  ConcatenateDimension=2
  Vector Concatenate2 : Concatenate
  Vector Concatenate3 : Concatenate
  R : Outport
  wires:
  Signal Specification2/1 -> Vector Concatenate1/2
  Signal Specification1/1 -> Vector Concatenate1/1
  Vector Concatenate2/1 -> Signal Specification1/1
  Vector Concatenate3/1 -> Signal Specification2/1
  angle (rad)/1 -> Trigonometric Function1/1
  Trigonometric Function1/2 -> Vector Concatenate2/1, Vector Concatenate3/2
  Vector Concatenate1/1 -> R/1
  Trigonometric Function1/1 -> Vector Concatenate2/2, Gain2/1
  Gain2/1 -> Vector Concatenate3/1

== system Marine_LocoMotive_UAV/UAV controller/Coupling/Coupling ==
  note: atan({U1.sin_psi-U2.cos_psi}/U3)
      |
      | asin{(U2.sin_psi+U1.cos_psi)/u1}
  U1 : Inport
  U3 : Inport  Port=2
  Add5 : Sum  Inputs=2
  Divide1 : Product  Inputs=*/
  Gain : Gain  Gain=m_u
  Product4 : Product
  Product5 : Product
  Saturation : Saturate  UpperLimit=LIMIT_uCMD_HEIGHT  LowerLimit=m_u*g*0.5
  Scope : Scope
  Scope1 : Scope
  Sqrt1 : Sqrt  SaturateOnIntegerOverflow=on
  Trigonometric Function2 : Trigonometry  Operator=atan
  u1 (N) : Outport
  phi_d (rad) : Outport  Port=2
  wires:
  U1/1 -> Divide1/1, Product4/2, Product4/1
  Divide1/1 -> Trigonometric Function2/1
  Trigonometric Function2/1 -> phi_d (rad)/1
  Product4/1 -> Add5/1, Scope/1
  Sqrt1/1 -> Gain/1
  Product5/1 -> Scope1/1, Add5/2
  Add5/1 -> Sqrt1/1
  U3/1 -> Divide1/2, Product5/1, Product5/2
  Saturation/1 -> u1 (N)/1
  Gain/1 -> Saturation/1

== system Marine_LocoMotive_UAV/UAV controller/Coupling/sat ==
  u : Inport
  Fcn1 : Fcn  Expr=LIMIT_CMD_PITCH*tanh(u(1)/LIMIT_CMD_PITCH)
  Manual Switch : ManualSwitch
  Saturation1 : Saturate  UpperLimit=LIMIT_CMD_PITCH  LowerLimit=-LIMIT_CMD_PITCH
  sat(u) : Outport
  wires:
  u/1 -> Fcn1/1, Saturation1/1
  Manual Switch/1 -> sat(u)/1
  Saturation1/1 -> Manual Switch/2
  Fcn1/1 -> Manual Switch/1

== system Marine_LocoMotive_UAV/UAV controller/Coupling /sat  ==
  u : Inport
  Fcn1 : Fcn  Expr=LIMIT_CMD_PITCH*tanh(u(1)/LIMIT_CMD_PITCH)
  Manual Switch : ManualSwitch
  Saturation1 : Saturate  UpperLimit=LIMIT_CMD_PITCH  LowerLimit=-LIMIT_CMD_PITCH
  sat(u) : Outport
  wires:
  u/1 -> Fcn1/1, Saturation1/1
  Manual Switch/1 -> sat(u)/1
  Saturation1/1 -> Manual Switch/2
  Fcn1/1 -> Manual Switch/1

== system Marine_LocoMotive_UAV/UAV controller/switch controllers/Smooth channel switching ==
  c1 : Inport
  switch : Inport  Port=2
  c2 : Inport  Port=3
  C1 transition : Subsystem
  C2 transition : Subsystem
  Delay : Delay  DelayLength=1
  Delay1 : Delay  DelayLength=1
  Logical Operator : Logic  Operator=NOT  AllPortsSameDT=off  OutDataTypeStr=boolean
  Mux3 : Mux  Inputs=3
  "c1,c2, u_out" : Scope
  c2 out if switch is 1 : Switch  Criteria=u2 > Threshold
  u_out : Outport
  wires:
  C2 transition/1(C2_trans) -> [c2_trans]  "C2 s"
  Logical Operator/1 -> C1 transition/2(switch)
  Delay1/1 -> C1 transition/3(C2_0)
  Delay/1 -> C2 transition/3(C1_0)
  Mux3/1 -> "c1,c2, u_out"/1
  switch/1 -> C2 transition/2(switch), Logical Operator/1, c2 out if switch is 1/2
  c2/1 -> C2 transition/1(C2), Mux3/2
  c2 out if switch is 1/1 -> u_out/1, Mux3/3  "out"
  c1/1 -> C1 transition/1(C1), Mux3/1
  C1 transition/1(C1_trans) -> [c1_trans]
  [c2_trans] -> Delay1/1
  [c1_trans] -> Delay/1
  [c1_trans] -> c2 out if switch is 1/3
  [c2_trans] -> c2 out if switch is 1/1

== system Marine_LocoMotive_UAV/UAV controller/switch controllers/smooth switch ==
  u 1 : Inport
  u 2 : Inport  Port=2
  switch : Inport  Port=3
  Constant : Constant
  Data Type Conversion : DataTypeConversion
  Low Pass Filter2 : DiscreteTransferFcn  Numerator=Bm_coup_LPF  Denominator=Am_coup_LPF
  Product : Product
  Product1 : Product
  Step1 : Step  SampleTime=0
  Subtract : Sum  Inputs=+-
  Sum : Sum  Inputs=|++
  "switch " : Scope
  y : Outport
  wires:
  Product/1 -> Sum/2
  Product1/1 -> Sum/1
  Low Pass Filter2/1 -> "switch "/1, Product/1, Subtract/2
  Data Type Conversion/1 -> Low Pass Filter2/1
  u 1/1 -> Product1/1
  u 2/1 -> Product/2
  switch/1 -> Data Type Conversion/1
  Sum/1 -> y/1
  Constant/1 -> Subtract/1
  Subtract/1 -> Product1/2

== system Marine_LocoMotive_UAV/UAV controller/u_a_Lyapunov/Subsystem ==
  In1 : Inport
  smothing : DiscreteTransferFcn  Numerator=Bm_coup_LPF  Denominator=Am_coup_LPF
  Out1 : Outport
  wires:
  smothing/1 -> Out1/1
  In1/1 -> smothing/1

== system Marine_LocoMotive_UAV/UAV controller/u_a_Lyapunov/Subsystem1 ==
  alpha_ref_ddot : Inport
  reset : Inport  Port=2
  Delay3 : Delay  Commented=on  DelayLength=1  InitialCondition=0
  Enabled Subsystem1 : Subsystem  Commented=on  TreatAsAtomicUnit=on
  Low Pass Filter5 : DiscreteTransferFcn  Numerator=Bm_rdeL_LPF  Denominator=Am_rdeL_LPF
  Switch : Switch  Commented=on  Criteria=u2 > Threshold
  alpha 0 : Subsystem  Commented=on  TreatAsAtomicUnit=on
  cond1 : Subsystem  Commented=on
  Out1 : Outport
  wires:
  reset/1 -> Delay3/1
  cond1/1(key) -> alpha 0/Trigger, Enabled Subsystem1/Enable, Switch/2
  Low Pass Filter5/1 -> Out1/1
  Delay3/1 -> Enabled Subsystem1/2(reset)
  alpha 0/1(Xu_init) -> Enabled Subsystem1/3(u0)
  Enabled Subsystem1/1(y) -> Switch/1
  alpha_ref_ddot/1 -> Low Pass Filter5/1, Switch/3, Enabled Subsystem1/1(u), alpha 0/1(X)

== system Marine_LocoMotive_UAV/UAV controller/u_r_V_Lyapunov buoy velocity/Smooth channel switching1 ==
  c1 : Inport
  switch : Inport  Port=2
  c2 : Inport  Port=3
  C1 transition : Subsystem
  C2 transition : Subsystem
  Delay : Delay  DelayLength=1
  Delay1 : Delay  DelayLength=1
  Logical Operator : Logic  Operator=NOT  AllPortsSameDT=off  OutDataTypeStr=boolean
  Mux3 : Mux  Inputs=3
  "c1,c2, u_out" : Scope
  c2 out if switch is 1 : Switch  Criteria=u2 > Threshold
  u_out : Outport
  wires:
  [c2_trans] -> c2 out if switch is 1/1
  [c1_trans] -> c2 out if switch is 1/3
  [c1_trans] -> Delay/1
  [c2_trans] -> Delay1/1
  C1 transition/1(C1_trans) -> [c1_trans]
  c1/1 -> Mux3/1, C1 transition/1(C1)
  c2 out if switch is 1/1 -> Mux3/3, u_out/1  "out"
  c2/1 -> Mux3/2, C2 transition/1(C2)
  switch/1 -> c2 out if switch is 1/2, Logical Operator/1, C2 transition/2(switch)
  Mux3/1 -> "c1,c2, u_out"/1
  Delay/1 -> C2 transition/3(C1_0)
  Delay1/1 -> C1 transition/3(C2_0)
  Logical Operator/1 -> C1 transition/2(switch)
  C2 transition/1(C2_trans) -> [c2_trans]  "C2 s"

== system Marine_LocoMotive_UAV/UAV controller/u_r_V_Lyapunov buoy velocity/Subsystem ==
  In1 : Inport
  smothing : DiscreteTransferFcn  Numerator=Bm_coup_LPF  Denominator=Am_coup_LPF
  Out1 : Outport
  wires:
  smothing/1 -> Out1/1
  In1/1 -> smothing/1

== system Marine_LocoMotive_UAV/UAV controller/u_r_V_Lyapunov buoy velocity/Subsystem1 ==
  In1 : Inport
  smothing : DiscreteTransferFcn  Numerator=Bm_coup_LPF  Denominator=Am_coup_LPF
  Out1 : Outport
  wires:
  In1/1 -> smothing/1
  smothing/1 -> Out1/1

== system Marine_LocoMotive_UAV/UAV controller/u_r_V_Lyapunov buoy velocity/smooth lower bound ==
  u : Inport
  Manual Switch : ManualSwitch
  Mux3 : Mux  Inputs=2
  Saturation1 : Saturate  UpperLimit=inf  LowerLimit=min_sf
  apply for lower bound only : Switch  Criteria=u2 > Threshold  Threshold=Amp_sf+min_sf
  sat : Scope
  saturation function : Fcn  Expr=Amp_sf*tanh((u(1)-(Amp_sf+min_sf))/(Amp_sf)) + (Amp_sf+min_sf)
  sat(u) : Outport
  wires:
  Manual Switch/1 -> sat(u)/1
  Saturation1/1 -> Manual Switch/2
  u/1 -> saturation function/1, apply for lower bound only/2, Mux3/1, apply for lower bound only/1, Saturation1/1
  saturation function/1 -> apply for lower bound only/3, Mux3/2
  Mux3/1 -> sat/1
  apply for lower bound only/1 -> Manual Switch/1

== system Marine_LocoMotive_UAV/UAV controller/u_r_p_Lyapunov radial position/Enabled Subsystem ==
  u : Inport
  reset : Inport  Port=2
  Enable : EnablePort
  Logical Operator : Logic  Operator=NOT  AllPortsSameDT=off  OutDataTypeStr=boolean
  Low Pass Filter5 : DiscreteTransferFcn  Numerator=Bm_reL_LPF  Denominator=Am_reL_LPF  ExternalReset=Level
      settings: InputPortMap=u0,r7
  y : Outport
  wires:
  u/1 -> Low Pass Filter5/1
  Low Pass Filter5/1 -> y/1
  Logical Operator/1 -> Low Pass Filter5/2
  reset/1 -> Logical Operator/1
